simulink model "fuzzy_test_Steven"  (R2014b)
settings: Solver=ode45  StartTime=0.0  StopTime=10.0  RelTol=1e-3
undefined symbols (not defined in the file): mfs, rls
libraries: simulink x1
settings Model: Creator=Steven  LastModifiedBy=Steven

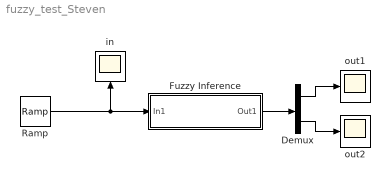
== system fuzzy_test_Steven ==
  Demux : Demux  Outputs=2
  Fuzzy Inference : Subsystem  mask(Fuzzy inference block){rls=rls, mfs=mfs, def=[1 3]}
      mask prompts: rls "Rule matrix:"; mfs "Membership functions matrix:"; def "Default output:"
      mask help:
      | MIN-MAX inference with
      |  fuzzy means defuzzification
      mask Help: Fuzzy inference block can be used as a direct fuzzy controller or as a fuzzy supervisor. For details on dialog parameters see INFER.
      mask Display: disp('Fuzzy Inference')
  Ramp : simulink/Sources/Ramp  slope=1  start=0  X0=0
  in : Scope
      settings: TimeRange=4  YMin=0  YMax=4  SaveName=ScopeData2
  out1 : Scope
      settings: TimeRange=4  YMin=0  YMax=4
  out2 : Scope
      settings: TimeRange=4  YMin=0  YMax=3
  wires:
  Fuzzy Inference/1(Out1) -> Demux/1
  Demux/1 -> out1/1
  Demux/2 -> out2/1
  Ramp/1 -> Fuzzy Inference/1(In1), in/1

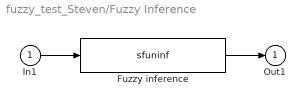
== system fuzzy_test_Steven/Fuzzy Inference ==
  In1 : Inport
  Fuzzy inference : S-Function  FunctionName=sfuninf  Parameters=rls, mfs, def  EnableBusSupport=off
  Out1 : Outport
  wires:
  In1/1 -> Fuzzy inference/1
  Fuzzy inference/1 -> Out1/1
